simulink model "Lab9_zadanie3"  (R2017a)
settings: Solver=FixedStepAuto  StartTime=0.0  StopTime=10.0  FixedStep=0.01  RelTol=1e-3
values from neighbouring files (symbols this model uses):
  a = (P1y - P2y) / (P1x - P2x)    (= 0.457251908397)    [Lab4.m]    (also in Lab8.m = 10; Lab9.m = 0.01)
  B = (pi*R2*R2)/(3*H2*H2)    (= 0.00337009933323)    [Lab2.m]    (also in Lab8.m = deltah20max / k; Lab9.m = 0.4; ModelDataNonlinear.m)
  delta = 0.005    [Lab9.m]
  ks = 10    [Lab9.m]
  Tm = Ts/(kr*ks)    (= 26.2488954345)    [Lab9.m]
  Ts = Ti    (= 17.823)    [Lab9.m]
libraries: cstblocks x3
settings Model: Creator=ishiguro  LastModifiedBy=ishiguro

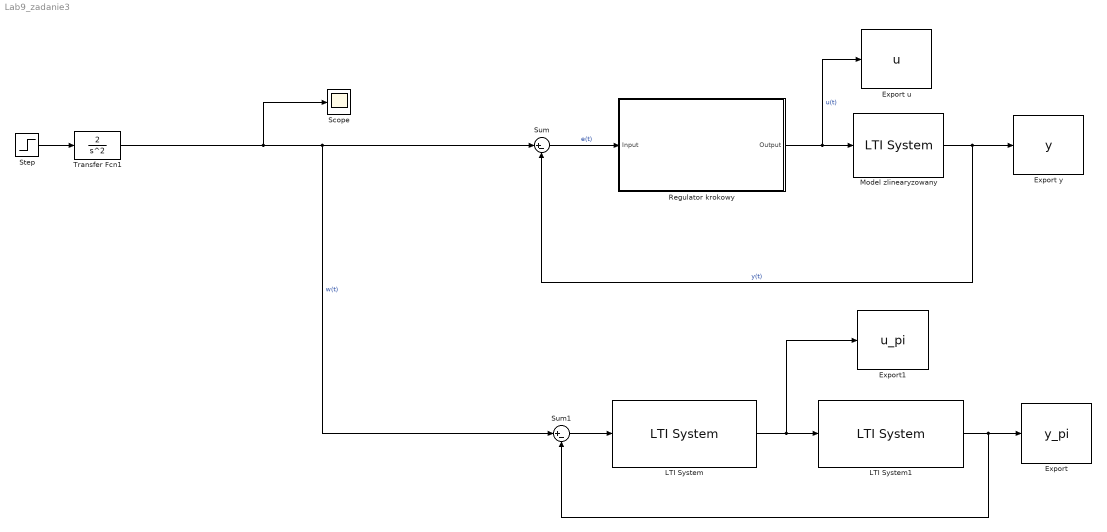
== system Lab9_zadanie3 ==
  Export : ToWorkspace  VariableName=y_pi  SaveFormat=Timeseries  SampleTime=-1
  Export u : ToWorkspace  VariableName=u  SaveFormat=Timeseries  SampleTime=-1
  Export y : ToWorkspace  VariableName=y  SaveFormat=Timeseries  SampleTime=-1
  Export1 : ToWorkspace  VariableName=u_pi  SaveFormat=Timeseries  SampleTime=-1
  LTI System : cstblocks/LTI System  sys=Kr  IC=[]
  LTI System1 : cstblocks/LTI System  sys=K  IC=[]
  Model zlinearyzowany : cstblocks/LTI System  sys=K  IC=[]
  "Regulator krokowy " : Subsystem
  Scope : Scope
  Step : Step  Time=0  SampleTime=0
  Sum : Sum  Inputs=|+-
  Sum1 : Sum  Inputs=|+-
  Transfer Fcn1 : TransferFcn  Numerator=[2]  Denominator=[1 0 0]
  wires:
  Sum/1 -> "Regulator krokowy "/1(Input)  "e(t)"
  "Regulator krokowy "/1(Output) -> Export u/1, Model zlinearyzowany/1  "u(t)"
  Model zlinearyzowany/1 -> Sum/2, Export y/1  "y(t)"
  LTI System1/1 -> Sum1/2, Export/1
  Sum1/1 -> LTI System/1
  LTI System/1 -> Export1/1, LTI System1/1
  Transfer Fcn1/1 -> Scope/1, Sum1/1, Sum/1  "w(t)"
  Step/1 -> Transfer Fcn1/1

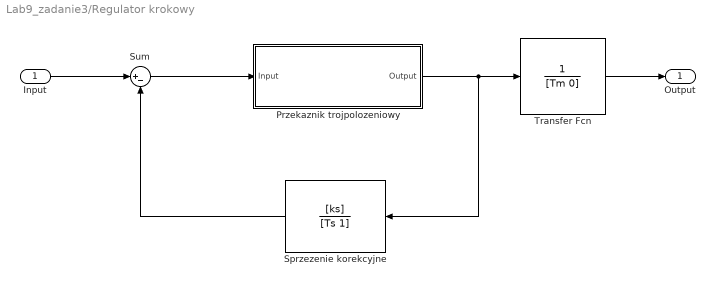
== system Lab9_zadanie3/Regulator krokowy  ==
  Input : Inport
  "Przekaznik trojpolozeniowy " : Subsystem
  Sprzezenie korekcyjne : TransferFcn  Numerator=[ks]  Denominator=[Ts 1]
  Sum : Sum  Inputs=|+-
  Transfer Fcn : TransferFcn  Denominator=[Tm 0]
  Output : Outport
  wires:
  "Przekaznik trojpolozeniowy "/1(Output) -> Sprzezenie korekcyjne/1, Transfer Fcn/1
  Sprzezenie korekcyjne/1 -> Sum/2
  Sum/1 -> "Przekaznik trojpolozeniowy "/1("Input ")
  Input/1 -> Sum/1
  Transfer Fcn/1 -> Output/1

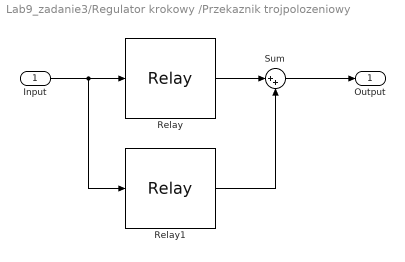
== system Lab9_zadanie3/Regulator krokowy /Przekaznik trojpolozeniowy  ==
  "Input " : Inport
  Relay : Relay  OnSwitchValue=-a  OffSwitchValue=-a-delta  OnOutputValue=0  OffOutputValue=-B
  Relay1 : Relay  OnSwitchValue=a+delta  OffSwitchValue=a  OnOutputValue=B
  Sum : Sum  Inputs=|++
  Output : Outport
  wires:
  "Input "/1 -> Relay1/1, Relay/1
  Relay1/1 -> Sum/2
  Relay/1 -> Sum/1
  Sum/1 -> Output/1
